simulink model "protocol_for_model_checking"  (R2021b)
settings: Solver=FixedStepAuto  StartTime=0.0  StopTime=10.0  RelTol=1e-3
settings Model: Creator=marco  LastModifiedBy=angelo
settings ConfigComp: DVTestSuiteOptimization=Auto  DVDetectOutOfBounds=on  DVModelReferenceHarness=on

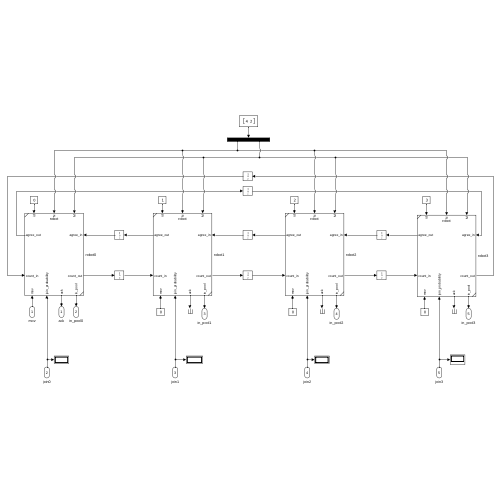
[thumbnail: Simulink's stored preview of the top-level diagram]
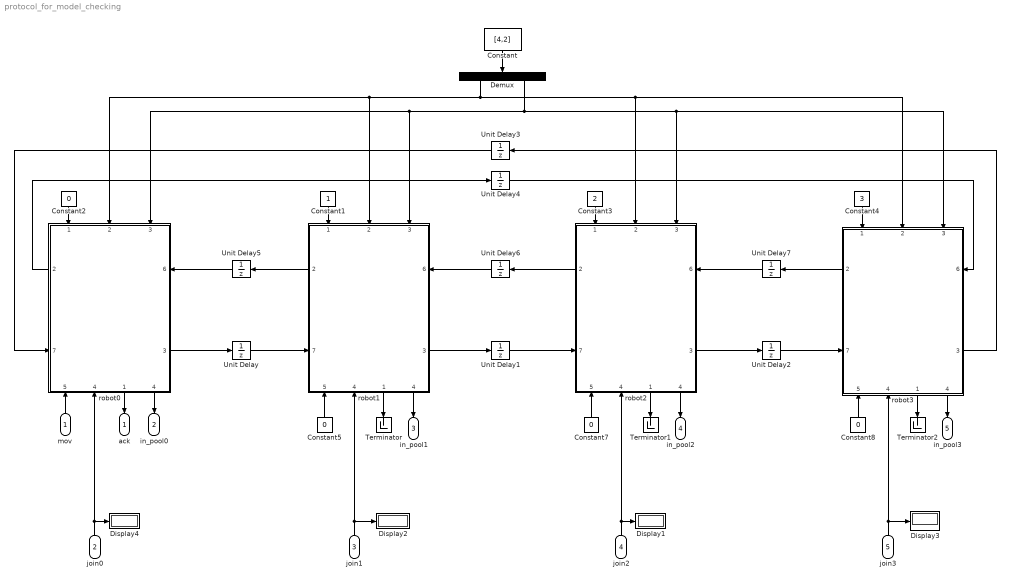
== system protocol_for_model_checking ==
  mov : Inport
  join0 : Inport  Port=2
  join1 : Inport  Port=3
  join2 : Inport  Port=4
  join3 : Inport  Port=5
  Constant : Constant  Value=[4,2]
  Constant1 : Constant
  Constant{2,5,7..8} (4 alike) : Constant  Value=0
  Constant3 : Constant  Value=2
  Constant4 : Constant  Value=3
  Demux : Demux  Outputs=2
  Display{1..4} (4 alike) : Display
  Terminator : Terminator
  Terminator1 : Terminator
  Terminator2 : Terminator
  Unit Delay{,1..7} (8 alike) : UnitDelay  SampleTime=-1  HasFrameUpgradeWarning=on
  robot{0..3} (4 alike) : Subsystem  ReferencedSubsystem=robot
      robot0 settings: PortSchema="{\"entries\":[{\"content\":{\"sides\":[{\"content\":{\"connectorIds\":[\"Out2\",\"In7\"]},\"type\":\"ConnectorPlacement.EquallySpacedRectSide\",\"uuid\":\"c2973ddf-8c1f-4294-82f9-250d4d64bc41\"},{\"content\":{\"connectorIds\":[\"In6\",\"Out3\"],\"side\":\"RIGHT\"},\"type\":\"ConnectorPlacement.EquallySpacedRectSide\",\"uuid\":\"34f58778-6b96-4f4c-9fc2-6c1c729063a8\"},{\"content\":{\"connectorIds\":[\"In1\",\"In2\",\"In3\"],\"side\":\"TOP\"},\"type\":\"ConnectorPlacement.EquallySpacedRectSide\",\"uuid\":\"80e910fc-ff47-444b-b672-e337659921ae\"},{\"content\":{\"connectorIds\":[\"In5\",\"In4\",\"Out1\",\"Out4\"],\"side\":\"BOTTOM\"},\"type\":\"ConnectorPlacement.EquallySpacedRectSide\",\"uuid\":\"4c5b4a6c-4ee5-43a5-b389-1d5635d4cbda\"}]},\"type\":\"ConnectorPlacement.EquallySpacedConnector\",\"uuid\":\"573bf93a-1f25-4267-812c-06cdd99b033a\"}],\"packageUris\":[\"http://schema.mathworks.com/mf0/Connector/R2020b\"],\"version\":\"1.0\"}"
      robot1 settings: PortSchema="{\"entries\":[{\"content\":{\"sides\":[{\"content\":{\"connectorIds\":[\"Out2\",\"In7\"]},\"type\":\"ConnectorPlacement.EquallySpacedRectSide\",\"uuid\":\"c2973ddf-8c1f-4294-82f9-250d4d64bc41\"},{\"content\":{\"connectorIds\":[\"In6\",\"Out3\"],\"side\":\"RIGHT\"},\"type\":\"ConnectorPlacement.EquallySpacedRectSide\",\"uuid\":\"34f58778-6b96-4f4c-9fc2-6c1c729063a8\"},{\"content\":{\"connectorIds\":[\"In1\",\"In2\",\"In3\"],\"side\":\"TOP\"},\"type\":\"ConnectorPlacement.EquallySpacedRectSide\",\"uuid\":\"80e910fc-ff47-444b-b672-e337659921ae\"},{\"content\":{\"connectorIds\":[\"In5\",\"In4\",\"Out1\",\"Out4\"],\"side\":\"BOTTOM\"},\"type\":\"ConnectorPlacement.EquallySpacedRectSide\",\"uuid\":\"e4e016b7-b76e-4e62-a0db-89e9df8dea8e\"}]},\"type\":\"ConnectorPlacement.EquallySpacedConnector\",\"uuid\":\"573bf93a-1f25-4267-812c-06cdd99b033a\"}],\"packageUris\":[\"http://schema.mathworks.com/mf0/Connector/R2020b\"],\"version\":\"1.0\"}"
      robot2 settings: PortSchema="{\"entries\":[{\"content\":{\"sides\":[{\"content\":{\"connectorIds\":[\"Out2\",\"In7\"]},\"type\":\"ConnectorPlacement.EquallySpacedRectSide\",\"uuid\":\"c2973ddf-8c1f-4294-82f9-250d4d64bc41\"},{\"content\":{\"connectorIds\":[\"In6\",\"Out3\"],\"side\":\"RIGHT\"},\"type\":\"ConnectorPlacement.EquallySpacedRectSide\",\"uuid\":\"34f58778-6b96-4f4c-9fc2-6c1c729063a8\"},{\"content\":{\"connectorIds\":[\"In1\",\"In2\",\"In3\"],\"side\":\"TOP\"},\"type\":\"ConnectorPlacement.EquallySpacedRectSide\",\"uuid\":\"80e910fc-ff47-444b-b672-e337659921ae\"},{\"content\":{\"connectorIds\":[\"In5\",\"In4\",\"Out1\",\"Out4\"],\"side\":\"BOTTOM\"},\"type\":\"ConnectorPlacement.EquallySpacedRectSide\",\"uuid\":\"2cd792df-4aad-4f2e-80f9-e48174994b0d\"}]},\"type\":\"ConnectorPlacement.EquallySpacedConnector\",\"uuid\":\"573bf93a-1f25-4267-812c-06cdd99b033a\"}],\"packageUris\":[\"http://schema.mathworks.com/mf0/Connector/R2020b\"],\"version\":\"1.0\"}"
      robot3 settings: PortSchema="{\"entries\":[{\"content\":{\"sides\":[{\"content\":{\"connectorIds\":[\"Out2\",\"In7\"]},\"type\":\"ConnectorPlacement.EquallySpacedRectSide\",\"uuid\":\"c2973ddf-8c1f-4294-82f9-250d4d64bc41\"},{\"content\":{\"connectorIds\":[\"In6\",\"Out3\"],\"side\":\"RIGHT\"},\"type\":\"ConnectorPlacement.EquallySpacedRectSide\",\"uuid\":\"34f58778-6b96-4f4c-9fc2-6c1c729063a8\"},{\"content\":{\"connectorIds\":[\"In1\",\"In2\",\"In3\"],\"side\":\"TOP\"},\"type\":\"ConnectorPlacement.EquallySpacedRectSide\",\"uuid\":\"80e910fc-ff47-444b-b672-e337659921ae\"},{\"content\":{\"connectorIds\":[\"In5\",\"In4\",\"Out1\",\"Out4\"],\"side\":\"BOTTOM\"},\"type\":\"ConnectorPlacement.EquallySpacedRectSide\",\"uuid\":\"e1d2a9a1-3695-4a7a-a698-108fcecfffe2\"}]},\"type\":\"ConnectorPlacement.EquallySpacedConnector\",\"uuid\":\"573bf93a-1f25-4267-812c-06cdd99b033a\"}],\"packageUris\":[\"http://schema.mathworks.com/mf0/Connector/R2020b\"],\"version\":\"1.0\"}"
  ack : Outport
  in_pool0 : Outport  Port=2
  in_pool1 : Outport  Port=3
  in_pool2 : Outport  Port=4
  in_pool3 : Outport  Port=5
  wires:
  Constant/1 -> Demux/1
  Constant2/1 -> robot0/1
  robot0/1 -> ack/1
  robot1/1 -> Terminator/1
  robot2/1 -> Terminator1/1
  robot3/1 -> Terminator2/1
  Constant1/1 -> robot1/1
  Constant3/1 -> robot2/1
  Constant4/1 -> robot3/1
  Constant5/1 -> robot1/5
  Constant7/1 -> robot2/5
  Constant8/1 -> robot3/5
  robot0/3 -> Unit Delay/1
  robot1/3 -> Unit Delay1/1
  robot2/3 -> Unit Delay2/1
  robot3/3 -> Unit Delay3/1
  robot1/2 -> Unit Delay5/1
  robot2/2 -> Unit Delay6/1
  robot3/2 -> Unit Delay7/1
  robot0/2 -> Unit Delay4/1
  Demux/1 -> robot2/2, robot3/2, robot1/2, robot0/2
  Demux/2 -> robot2/3, robot3/3, robot1/3, robot0/3
  join1/1 -> robot1/4, Display2/1
  join2/1 -> robot2/4, Display1/1
  Unit Delay/1 -> robot1/7
  Unit Delay1/1 -> robot2/7
  Unit Delay2/1 -> robot3/7
  Unit Delay3/1 -> robot0/7
  Unit Delay4/1 -> robot3/6
  Unit Delay5/1 -> robot0/6
  Unit Delay6/1 -> robot1/6
  Unit Delay7/1 -> robot2/6
  join0/1 -> robot0/4, Display4/1
  mov/1 -> robot0/5
  join3/1 -> robot3/4, Display3/1
  robot0/4 -> in_pool0/1
  robot1/4 -> in_pool1/1
  robot2/4 -> in_pool2/1
  robot3/4 -> in_pool3/1
